simulink model "String3_Diode"  (R2023b)
settings: Solver=VariableStepAuto  StartTime=0.0  StopTime=1  FixedStep=Ts_Power  MinStep=0.0025  RelTol=1e-4
PreLoadFcn:
  | Ts_Power=5e-4;
  | Slope_Vdc=1;
InitFcn:
  | Ts_Power=50e-6;
  | Tc=1e-5;%break algebraic loop time constant
StopFcn:
  | if exist('I','var') && exist('V','var')
  |    figure(1)
  |    clf
  |    n=find(I>=0);
  |    n=n(end);
  |    Vglobal=V(1:n);
  |    Iglobal=I(1:n);
  | 
  | 
  |    Pglobal=Vglobal.*Iglobal;
  |    n=find(Pglobal==max(Pglobal));
  |    Pmax=Pglobal(n);
  |    Vmp=Vglobal(n);
  |    Imp=Iglobal(n);
  | 
  | 
  |    subplot(211)
  |    plot(Vglobal, Iglobal,Vmp,Imp,'or')
  |    ylabel('Current (A)')
  |    title(sprintf('Global I-V & P-V characteristics\n %s' ,ModuleName))
  | 
  | 
  |    subplot(212)
  |    plot(Vglobal, Pglobal,Vmp,Pmax,'or')
  |    ylabel('Power (W)')
  |    xlabel('Voltage (V)')
  | end
model workspace (MAT data in the model file):
  slope_Vdc = 3.0848387096
values from neighbouring files (symbols this model uses):
  Slope_Vdc_string3 = 90 * 0.77    (= 69.3)    [totPower.m]
libraries: spsPVArrayLib x90, spsVariableResistorLib x90, spsDiodeLib x20, spsCurrentMeasurementLib x1, spsVoltageMeasurementLib x1, spsControlledVoltageSourceLib x1, simulink x1, spspowerguiLib x1
(part 4 of 5)

== system String3_Diode/Subsystem17/PV10 ==
  Irr : Inport
  1PΩ : Constant  Value=1e15
  PV1 : spsPVArrayLib/PV Array  Npar=1  Nser=1  PlotType=array @ 25 deg.C & specified irradiances  S_vec="[ 1000  500  100 ]"  Temp_C_vec="[ 45 25  ]"  ModuleName=User-defined  PlotWhenSelected=off  Pm=3.8061  Ncell=1  Voc=0.7315  Isc=6.41  Vm=0.626  Im=6.08  beta_Voc_pc=-0.2256195755  alpha_Isc_pc=0.04692556634  beta_Voc=-0.0016504  alpha_Isc=0.0030079  IL=6.4137  I0=6.5578e-13  nI=0.95237  Rsh=7.312  Rs=0.0042689  RobustModel=on  RobustCellTemperature=25  BAL=on  Tc=1e-5  Tfilter=5e-5
  Terminator1 : Terminator
  Variable Resistor2 : spsVariableResistorLib/Variable Resistor  Rabsmin=1e-3
      settings: LibrarySourceBlock=sps_lib/Passives/Variable Resistor
  + : PMIOPort  Side=Left
  - : PMIOPort  Port=2  Side=Right
  wires:
  Irr/1 -> PV1/1
  1PΩ/1 -> Variable Resistor2/1
  PV1/1 -> Terminator1/1
  connections:
  PV1/RConn2 -- -/RConn1 -- Variable Resistor2/RConn1
  +/RConn1 -- Variable Resistor2/LConn1 -- PV1/RConn1

== system String3_Diode/Subsystem17/PV11 ==
  Irr : Inport
  1PΩ : Constant  Value=1e15
  PV2 : spsPVArrayLib/PV Array  Npar=1  Nser=1  PlotType=array @ 25 deg.C & specified irradiances  S_vec="[ 1000  500  100 ]"  Temp_C_vec="[ 45 25  ]"  ModuleName=User-defined  PlotWhenSelected=off  Pm=3.8061  Ncell=1  Voc=0.7315  Isc=6.41  Vm=0.626  Im=6.08  beta_Voc_pc=-0.2256195755  alpha_Isc_pc=0.04692556634  beta_Voc=-0.0016504  alpha_Isc=0.0030079  IL=6.4137  I0=6.5578e-13  nI=0.95237  Rsh=7.312  Rs=0.0042689  RobustModel=on  RobustCellTemperature=25  BAL=on  Tc=1e-5  Tfilter=5e-5
  Terminator1 : Terminator
  Variable Resistor2 : spsVariableResistorLib/Variable Resistor  Rabsmin=1e-3
      settings: LibrarySourceBlock=sps_lib/Passives/Variable Resistor
  + : PMIOPort  Side=Left
  - : PMIOPort  Port=2  Side=Right
  wires:
  Irr/1 -> PV2/1
  1PΩ/1 -> Variable Resistor2/1
  PV2/1 -> Terminator1/1
  connections:
  -/RConn1 -- Variable Resistor2/RConn1 -- PV2/RConn2
  +/RConn1 -- Variable Resistor2/LConn1 -- PV2/RConn1

== system String3_Diode/Subsystem17/PV2 ==
  Irr : Inport
  1PΩ : Constant  Value=1e15
  PV1 : spsPVArrayLib/PV Array  Npar=1  Nser=1  PlotType=array @ 25 deg.C & specified irradiances  S_vec="[ 1000  500  100 ]"  Temp_C_vec="[ 45 25  ]"  ModuleName=User-defined  PlotWhenSelected=off  Pm=3.8061  Ncell=1  Voc=0.7315  Isc=6.41  Vm=0.626  Im=6.08  beta_Voc_pc=-0.2256195755  alpha_Isc_pc=0.04692556634  beta_Voc=-0.0016504  alpha_Isc=0.0030079  IL=6.4137  I0=6.5578e-13  nI=0.95237  Rsh=7.312  Rs=0.0042689  RobustModel=on  RobustCellTemperature=25  BAL=on  Tc=1e-5  Tfilter=5e-5
  Terminator1 : Terminator
  Variable Resistor2 : spsVariableResistorLib/Variable Resistor  Rabsmin=1e-3
      settings: LibrarySourceBlock=sps_lib/Passives/Variable Resistor
  + : PMIOPort  Side=Left
  - : PMIOPort  Port=2  Side=Right
  wires:
  Irr/1 -> PV1/1
  1PΩ/1 -> Variable Resistor2/1
  PV1/1 -> Terminator1/1
  connections:
  PV1/RConn2 -- -/RConn1 -- Variable Resistor2/RConn1
  +/RConn1 -- Variable Resistor2/LConn1 -- PV1/RConn1

== system String3_Diode/Subsystem17/PV3 ==
  Irr : Inport
  1PΩ : Constant  Value=1e15
  PV1 : spsPVArrayLib/PV Array  Npar=1  Nser=1  PlotType=array @ 25 deg.C & specified irradiances  S_vec="[ 1000  500  100 ]"  Temp_C_vec="[ 45 25  ]"  ModuleName=User-defined  PlotWhenSelected=off  Pm=3.8061  Ncell=1  Voc=0.7315  Isc=6.41  Vm=0.626  Im=6.08  beta_Voc_pc=-0.2256195755  alpha_Isc_pc=0.04692556634  beta_Voc=-0.0016504  alpha_Isc=0.0030079  IL=6.4137  I0=6.5578e-13  nI=0.95237  Rsh=7.312  Rs=0.0042689  RobustModel=on  RobustCellTemperature=25  BAL=on  Tc=1e-5  Tfilter=5e-5
  Terminator1 : Terminator
  Variable Resistor2 : spsVariableResistorLib/Variable Resistor  Rabsmin=1e-3
      settings: LibrarySourceBlock=sps_lib/Passives/Variable Resistor
  + : PMIOPort  Side=Left
  - : PMIOPort  Port=2  Side=Right
  wires:
  Irr/1 -> PV1/1
  1PΩ/1 -> Variable Resistor2/1
  PV1/1 -> Terminator1/1
  connections:
  PV1/RConn2 -- -/RConn1 -- Variable Resistor2/RConn1
  +/RConn1 -- Variable Resistor2/LConn1 -- PV1/RConn1

== system String3_Diode/Subsystem18/PV1 ==
  Irr : Inport
  1PΩ : Constant  Value=1e15
  PV2 : spsPVArrayLib/PV Array  Npar=1  Nser=1  PlotType=array @ 25 deg.C & specified irradiances  S_vec="[ 1000  500  100 ]"  Temp_C_vec="[ 45 25  ]"  ModuleName=User-defined  PlotWhenSelected=off  Pm=3.8061  Ncell=1  Voc=0.7315  Isc=6.41  Vm=0.626  Im=6.08  beta_Voc_pc=-0.2256195755  alpha_Isc_pc=0.04692556634  beta_Voc=-0.0016504  alpha_Isc=0.0030079  IL=6.4137  I0=6.5578e-13  nI=0.95237  Rsh=7.312  Rs=0.0042689  RobustModel=on  RobustCellTemperature=25  BAL=on  Tc=1e-5  Tfilter=5e-5
  Terminator1 : Terminator
  Variable Resistor2 : spsVariableResistorLib/Variable Resistor  Rabsmin=1e-3
      settings: LibrarySourceBlock=sps_lib/Passives/Variable Resistor
  + : PMIOPort  Side=Left
  - : PMIOPort  Port=2  Side=Right
  wires:
  Irr/1 -> PV2/1
  1PΩ/1 -> Variable Resistor2/1
  PV2/1 -> Terminator1/1
  connections:
  -/RConn1 -- Variable Resistor2/RConn1 -- PV2/RConn2
  +/RConn1 -- Variable Resistor2/LConn1 -- PV2/RConn1

== system String3_Diode/Subsystem18/PV2 ==
  Irr : Inport
  1PΩ : Constant  Value=1e15
  PV2 : spsPVArrayLib/PV Array  Npar=1  Nser=1  PlotType=array @ 25 deg.C & specified irradiances  S_vec="[ 1000  500  100 ]"  Temp_C_vec="[ 45 25  ]"  ModuleName=User-defined  PlotWhenSelected=off  Pm=3.8061  Ncell=1  Voc=0.7315  Isc=6.41  Vm=0.626  Im=6.08  beta_Voc_pc=-0.2256195755  alpha_Isc_pc=0.04692556634  beta_Voc=-0.0016504  alpha_Isc=0.0030079  IL=6.4137  I0=6.5578e-13  nI=0.95237  Rsh=7.312  Rs=0.0042689  RobustModel=on  RobustCellTemperature=25  BAL=on  Tc=1e-5  Tfilter=5e-5
  Terminator1 : Terminator
  Variable Resistor2 : spsVariableResistorLib/Variable Resistor  Rabsmin=1e-3
      settings: LibrarySourceBlock=sps_lib/Passives/Variable Resistor
  + : PMIOPort  Side=Left
  - : PMIOPort  Port=2  Side=Right
  wires:
  Irr/1 -> PV2/1
  1PΩ/1 -> Variable Resistor2/1
  PV2/1 -> Terminator1/1
  connections:
  -/RConn1 -- Variable Resistor2/RConn1 -- PV2/RConn2
  +/RConn1 -- Variable Resistor2/LConn1 -- PV2/RConn1

== system String3_Diode/Subsystem18/PV3 ==
  Irr : Inport
  1PΩ : Constant  Value=1e15
  PV2 : spsPVArrayLib/PV Array  Npar=1  Nser=1  PlotType=array @ 25 deg.C & specified irradiances  S_vec="[ 1000  500  100 ]"  Temp_C_vec="[ 45 25  ]"  ModuleName=User-defined  PlotWhenSelected=off  Pm=3.8061  Ncell=1  Voc=0.7315  Isc=6.41  Vm=0.626  Im=6.08  beta_Voc_pc=-0.2256195755  alpha_Isc_pc=0.04692556634  beta_Voc=-0.0016504  alpha_Isc=0.0030079  IL=6.4137  I0=6.5578e-13  nI=0.95237  Rsh=7.312  Rs=0.0042689  RobustModel=on  RobustCellTemperature=25  BAL=on  Tc=1e-5  Tfilter=5e-5
  Terminator1 : Terminator
  Variable Resistor2 : spsVariableResistorLib/Variable Resistor  Rabsmin=1e-3
      settings: LibrarySourceBlock=sps_lib/Passives/Variable Resistor
  + : PMIOPort  Side=Left
  - : PMIOPort  Port=2  Side=Right
  wires:
  Irr/1 -> PV2/1
  1PΩ/1 -> Variable Resistor2/1
  PV2/1 -> Terminator1/1
  connections:
  -/RConn1 -- PV2/RConn2 -- Variable Resistor2/RConn1
  +/RConn1 -- PV2/RConn1 -- Variable Resistor2/LConn1

== system String3_Diode/Subsystem18/PV4 ==
  Irr : Inport
  1PΩ : Constant  Value=1e15
  PV2 : spsPVArrayLib/PV Array  Npar=1  Nser=1  PlotType=array @ 25 deg.C & specified irradiances  S_vec="[ 1000  500  100 ]"  Temp_C_vec="[ 45 25  ]"  ModuleName=User-defined  PlotWhenSelected=off  Pm=3.8061  Ncell=1  Voc=0.7315  Isc=6.41  Vm=0.626  Im=6.08  beta_Voc_pc=-0.2256195755  alpha_Isc_pc=0.04692556634  beta_Voc=-0.0016504  alpha_Isc=0.0030079  IL=6.4137  I0=6.5578e-13  nI=0.95237  Rsh=7.312  Rs=0.0042689  RobustModel=on  RobustCellTemperature=25  BAL=on  Tc=1e-5  Tfilter=5e-5
  Terminator1 : Terminator
  Variable Resistor2 : spsVariableResistorLib/Variable Resistor  Rabsmin=1e-3
      settings: LibrarySourceBlock=sps_lib/Passives/Variable Resistor
  + : PMIOPort  Side=Left
  - : PMIOPort  Port=2  Side=Right
  wires:
  Irr/1 -> PV2/1
  1PΩ/1 -> Variable Resistor2/1
  PV2/1 -> Terminator1/1
  connections:
  -/RConn1 -- Variable Resistor2/RConn1 -- PV2/RConn2
  +/RConn1 -- Variable Resistor2/LConn1 -- PV2/RConn1

== system String3_Diode/Subsystem19/PV1 ==
  Irr : Inport
  1PΩ : Constant  Value=1e15
  PV2 : spsPVArrayLib/PV Array  Npar=1  Nser=1  PlotType=array @ 25 deg.C & specified irradiances  S_vec="[ 1000  500  100 ]"  Temp_C_vec="[ 45 25  ]"  ModuleName=User-defined  PlotWhenSelected=off  Pm=3.8061  Ncell=1  Voc=0.7315  Isc=6.41  Vm=0.626  Im=6.08  beta_Voc_pc=-0.2256195755  alpha_Isc_pc=0.04692556634  beta_Voc=-0.0016504  alpha_Isc=0.0030079  IL=6.4137  I0=6.5578e-13  nI=0.95237  Rsh=7.312  Rs=0.0042689  RobustModel=on  RobustCellTemperature=25  BAL=on  Tc=1e-5  Tfilter=5e-5
  Terminator1 : Terminator
  Variable Resistor2 : spsVariableResistorLib/Variable Resistor  Rabsmin=1e-3
      settings: LibrarySourceBlock=sps_lib/Passives/Variable Resistor
  + : PMIOPort  Side=Left
  - : PMIOPort  Port=2  Side=Right
  wires:
  Irr/1 -> PV2/1
  1PΩ/1 -> Variable Resistor2/1
  PV2/1 -> Terminator1/1
  connections:
  -/RConn1 -- Variable Resistor2/RConn1 -- PV2/RConn2
  +/RConn1 -- Variable Resistor2/LConn1 -- PV2/RConn1

== system String3_Diode/Subsystem19/PV2 ==
  Irr : Inport
  1PΩ : Constant  Value=1e15
  PV2 : spsPVArrayLib/PV Array  Npar=1  Nser=1  PlotType=array @ 25 deg.C & specified irradiances  S_vec="[ 1000  500  100 ]"  Temp_C_vec="[ 45 25  ]"  ModuleName=User-defined  PlotWhenSelected=off  Pm=3.8061  Ncell=1  Voc=0.7315  Isc=6.41  Vm=0.626  Im=6.08  beta_Voc_pc=-0.2256195755  alpha_Isc_pc=0.04692556634  beta_Voc=-0.0016504  alpha_Isc=0.0030079  IL=6.4137  I0=6.5578e-13  nI=0.95237  Rsh=7.312  Rs=0.0042689  RobustModel=on  RobustCellTemperature=25  BAL=on  Tc=1e-5  Tfilter=5e-5
  Terminator1 : Terminator
  Variable Resistor2 : spsVariableResistorLib/Variable Resistor  Rabsmin=1e-3
      settings: LibrarySourceBlock=sps_lib/Passives/Variable Resistor
  + : PMIOPort  Side=Left
  - : PMIOPort  Port=2  Side=Right
  wires:
  Irr/1 -> PV2/1
  1PΩ/1 -> Variable Resistor2/1
  PV2/1 -> Terminator1/1
  connections:
  -/RConn1 -- Variable Resistor2/RConn1 -- PV2/RConn2
  +/RConn1 -- Variable Resistor2/LConn1 -- PV2/RConn1

== system String3_Diode/Subsystem19/PV3 ==
  Irr : Inport
  1PΩ : Constant  Value=1e15
  PV2 : spsPVArrayLib/PV Array  Npar=1  Nser=1  PlotType=array @ 25 deg.C & specified irradiances  S_vec="[ 1000  500  100 ]"  Temp_C_vec="[ 45 25  ]"  ModuleName=User-defined  PlotWhenSelected=off  Pm=3.8061  Ncell=1  Voc=0.7315  Isc=6.41  Vm=0.626  Im=6.08  beta_Voc_pc=-0.2256195755  alpha_Isc_pc=0.04692556634  beta_Voc=-0.0016504  alpha_Isc=0.0030079  IL=6.4137  I0=6.5578e-13  nI=0.95237  Rsh=7.312  Rs=0.0042689  RobustModel=on  RobustCellTemperature=25  BAL=on  Tc=1e-5  Tfilter=5e-5
  Terminator1 : Terminator
  Variable Resistor2 : spsVariableResistorLib/Variable Resistor  Rabsmin=1e-3
      settings: LibrarySourceBlock=sps_lib/Passives/Variable Resistor
  + : PMIOPort  Side=Left
  - : PMIOPort  Port=2  Side=Right
  wires:
  Irr/1 -> PV2/1
  1PΩ/1 -> Variable Resistor2/1
  PV2/1 -> Terminator1/1
  connections:
  -/RConn1 -- PV2/RConn2 -- Variable Resistor2/RConn1
  +/RConn1 -- PV2/RConn1 -- Variable Resistor2/LConn1

== system String3_Diode/Subsystem19/PV4 ==
  Irr : Inport
  1PΩ : Constant  Value=1e15
  PV2 : spsPVArrayLib/PV Array  Npar=1  Nser=1  PlotType=array @ 25 deg.C & specified irradiances  S_vec="[ 1000  500  100 ]"  Temp_C_vec="[ 45 25  ]"  ModuleName=User-defined  PlotWhenSelected=off  Pm=3.8061  Ncell=1  Voc=0.7315  Isc=6.41  Vm=0.626  Im=6.08  beta_Voc_pc=-0.2256195755  alpha_Isc_pc=0.04692556634  beta_Voc=-0.0016504  alpha_Isc=0.0030079  IL=6.4137  I0=6.5578e-13  nI=0.95237  Rsh=7.312  Rs=0.0042689  RobustModel=on  RobustCellTemperature=25  BAL=on  Tc=1e-5  Tfilter=5e-5
  Terminator1 : Terminator
  Variable Resistor2 : spsVariableResistorLib/Variable Resistor  Rabsmin=1e-3
      settings: LibrarySourceBlock=sps_lib/Passives/Variable Resistor
  + : PMIOPort  Side=Left
  - : PMIOPort  Port=2  Side=Right
  wires:
  Irr/1 -> PV2/1
  1PΩ/1 -> Variable Resistor2/1
  PV2/1 -> Terminator1/1
  connections:
  -/RConn1 -- Variable Resistor2/RConn1 -- PV2/RConn2
  +/RConn1 -- Variable Resistor2/LConn1 -- PV2/RConn1

== system String3_Diode/Subsystem20/PV1 ==
  Irr : Inport
  1PΩ : Constant  Value=1e15
  PV2 : spsPVArrayLib/PV Array  Npar=1  Nser=1  PlotType=array @ 25 deg.C & specified irradiances  S_vec="[ 1000  500  100 ]"  Temp_C_vec="[ 45 25  ]"  ModuleName=User-defined  PlotWhenSelected=off  Pm=3.8061  Ncell=1  Voc=0.7315  Isc=6.41  Vm=0.626  Im=6.08  beta_Voc_pc=-0.2256195755  alpha_Isc_pc=0.04692556634  beta_Voc=-0.0016504  alpha_Isc=0.0030079  IL=6.4137  I0=6.5578e-13  nI=0.95237  Rsh=7.312  Rs=0.0042689  RobustModel=on  RobustCellTemperature=25  BAL=on  Tc=1e-5  Tfilter=5e-5
  Terminator1 : Terminator
  Variable Resistor2 : spsVariableResistorLib/Variable Resistor  Rabsmin=1e-3
      settings: LibrarySourceBlock=sps_lib/Passives/Variable Resistor
  + : PMIOPort  Side=Left
  - : PMIOPort  Port=2  Side=Right
  wires:
  Irr/1 -> PV2/1
  1PΩ/1 -> Variable Resistor2/1
  PV2/1 -> Terminator1/1
  connections:
  -/RConn1 -- Variable Resistor2/RConn1 -- PV2/RConn2
  +/RConn1 -- Variable Resistor2/LConn1 -- PV2/RConn1

== system String3_Diode/Subsystem20/PV2 ==
  Irr : Inport
  1PΩ : Constant  Value=1e15
  PV2 : spsPVArrayLib/PV Array  Npar=1  Nser=1  PlotType=array @ 25 deg.C & specified irradiances  S_vec="[ 1000  500  100 ]"  Temp_C_vec="[ 45 25  ]"  ModuleName=User-defined  PlotWhenSelected=off  Pm=3.8061  Ncell=1  Voc=0.7315  Isc=6.41  Vm=0.626  Im=6.08  beta_Voc_pc=-0.2256195755  alpha_Isc_pc=0.04692556634  beta_Voc=-0.0016504  alpha_Isc=0.0030079  IL=6.4137  I0=6.5578e-13  nI=0.95237  Rsh=7.312  Rs=0.0042689  RobustModel=on  RobustCellTemperature=25  BAL=on  Tc=1e-5  Tfilter=5e-5
  Terminator1 : Terminator
  Variable Resistor2 : spsVariableResistorLib/Variable Resistor  Rabsmin=1e-3
      settings: LibrarySourceBlock=sps_lib/Passives/Variable Resistor
  + : PMIOPort  Side=Left
  - : PMIOPort  Port=2  Side=Right
  wires:
  Irr/1 -> PV2/1
  1PΩ/1 -> Variable Resistor2/1
  PV2/1 -> Terminator1/1
  connections:
  -/RConn1 -- Variable Resistor2/RConn1 -- PV2/RConn2
  +/RConn1 -- Variable Resistor2/LConn1 -- PV2/RConn1

== system String3_Diode/Subsystem20/PV3 ==
  Irr : Inport
  1PΩ : Constant  Value=1e15
  PV2 : spsPVArrayLib/PV Array  Npar=1  Nser=1  PlotType=array @ 25 deg.C & specified irradiances  S_vec="[ 1000  500  100 ]"  Temp_C_vec="[ 45 25  ]"  ModuleName=User-defined  PlotWhenSelected=off  Pm=3.8061  Ncell=1  Voc=0.7315  Isc=6.41  Vm=0.626  Im=6.08  beta_Voc_pc=-0.2256195755  alpha_Isc_pc=0.04692556634  beta_Voc=-0.0016504  alpha_Isc=0.0030079  IL=6.4137  I0=6.5578e-13  nI=0.95237  Rsh=7.312  Rs=0.0042689  RobustModel=on  RobustCellTemperature=25  BAL=on  Tc=1e-5  Tfilter=5e-5
  Terminator1 : Terminator
  Variable Resistor2 : spsVariableResistorLib/Variable Resistor  Rabsmin=1e-3
      settings: LibrarySourceBlock=sps_lib/Passives/Variable Resistor
  + : PMIOPort  Side=Left
  - : PMIOPort  Port=2  Side=Right
  wires:
  Irr/1 -> PV2/1
  1PΩ/1 -> Variable Resistor2/1
  PV2/1 -> Terminator1/1
  connections:
  -/RConn1 -- PV2/RConn2 -- Variable Resistor2/RConn1
  +/RConn1 -- PV2/RConn1 -- Variable Resistor2/LConn1

== system String3_Diode/Subsystem20/PV4 ==
  Irr : Inport
  1PΩ : Constant  Value=1e15
  PV2 : spsPVArrayLib/PV Array  Npar=1  Nser=1  PlotType=array @ 25 deg.C & specified irradiances  S_vec="[ 1000  500  100 ]"  Temp_C_vec="[ 45 25  ]"  ModuleName=User-defined  PlotWhenSelected=off  Pm=3.8061  Ncell=1  Voc=0.7315  Isc=6.41  Vm=0.626  Im=6.08  beta_Voc_pc=-0.2256195755  alpha_Isc_pc=0.04692556634  beta_Voc=-0.0016504  alpha_Isc=0.0030079  IL=6.4137  I0=6.5578e-13  nI=0.95237  Rsh=7.312  Rs=0.0042689  RobustModel=on  RobustCellTemperature=25  BAL=on  Tc=1e-5  Tfilter=5e-5
  Terminator1 : Terminator
  Variable Resistor2 : spsVariableResistorLib/Variable Resistor  Rabsmin=1e-3
      settings: LibrarySourceBlock=sps_lib/Passives/Variable Resistor
  + : PMIOPort  Side=Left
  - : PMIOPort  Port=2  Side=Right
  wires:
  Irr/1 -> PV2/1
  1PΩ/1 -> Variable Resistor2/1
  PV2/1 -> Terminator1/1
  connections:
  -/RConn1 -- Variable Resistor2/RConn1 -- PV2/RConn2
  +/RConn1 -- Variable Resistor2/LConn1 -- PV2/RConn1

== system String3_Diode/Subsystem25/PV1 ==
  Irr : Inport
  1PΩ : Constant  Value=1e15
  PV2 : spsPVArrayLib/PV Array  Npar=1  Nser=1  PlotType=array @ 25 deg.C & specified irradiances  S_vec="[ 1000  500  100 ]"  Temp_C_vec="[ 45 25  ]"  ModuleName=User-defined  PlotWhenSelected=off  Pm=3.8061  Ncell=1  Voc=0.7315  Isc=6.41  Vm=0.626  Im=6.08  beta_Voc_pc=-0.2256195755  alpha_Isc_pc=0.04692556634  beta_Voc=-0.0016504  alpha_Isc=0.0030079  IL=6.4137  I0=6.5578e-13  nI=0.95237  Rsh=7.312  Rs=0.0042689  RobustModel=on  RobustCellTemperature=25  BAL=on  Tc=1e-5  Tfilter=5e-5
  Terminator1 : Terminator
  Variable Resistor2 : spsVariableResistorLib/Variable Resistor  Rabsmin=1e-3
      settings: LibrarySourceBlock=sps_lib/Passives/Variable Resistor
  + : PMIOPort  Side=Left
  - : PMIOPort  Port=2  Side=Right
  wires:
  Irr/1 -> PV2/1
  1PΩ/1 -> Variable Resistor2/1
  PV2/1 -> Terminator1/1
  connections:
  -/RConn1 -- Variable Resistor2/RConn1 -- PV2/RConn2
  +/RConn1 -- Variable Resistor2/LConn1 -- PV2/RConn1

== system String3_Diode/Subsystem25/PV2 ==
  Irr : Inport
  1PΩ : Constant  Value=1e15
  PV2 : spsPVArrayLib/PV Array  Npar=1  Nser=1  PlotType=array @ 25 deg.C & specified irradiances  S_vec="[ 1000  500  100 ]"  Temp_C_vec="[ 45 25  ]"  ModuleName=User-defined  PlotWhenSelected=off  Pm=3.8061  Ncell=1  Voc=0.7315  Isc=6.41  Vm=0.626  Im=6.08  beta_Voc_pc=-0.2256195755  alpha_Isc_pc=0.04692556634  beta_Voc=-0.0016504  alpha_Isc=0.0030079  IL=6.4137  I0=6.5578e-13  nI=0.95237  Rsh=7.312  Rs=0.0042689  RobustModel=on  RobustCellTemperature=25  BAL=on  Tc=1e-5  Tfilter=5e-5
  Terminator1 : Terminator
  Variable Resistor2 : spsVariableResistorLib/Variable Resistor  Rabsmin=1e-3
      settings: LibrarySourceBlock=sps_lib/Passives/Variable Resistor
  + : PMIOPort  Side=Left
  - : PMIOPort  Port=2  Side=Right
  wires:
  Irr/1 -> PV2/1
  1PΩ/1 -> Variable Resistor2/1
  PV2/1 -> Terminator1/1
  connections:
  -/RConn1 -- Variable Resistor2/RConn1 -- PV2/RConn2
  +/RConn1 -- Variable Resistor2/LConn1 -- PV2/RConn1

== system String3_Diode/Subsystem25/PV3 ==
  Irr : Inport
  1PΩ : Constant  Value=1e15
  PV2 : spsPVArrayLib/PV Array  Npar=1  Nser=1  PlotType=array @ 25 deg.C & specified irradiances  S_vec="[ 1000  500  100 ]"  Temp_C_vec="[ 45 25  ]"  ModuleName=User-defined  PlotWhenSelected=off  Pm=3.8061  Ncell=1  Voc=0.7315  Isc=6.41  Vm=0.626  Im=6.08  beta_Voc_pc=-0.2256195755  alpha_Isc_pc=0.04692556634  beta_Voc=-0.0016504  alpha_Isc=0.0030079  IL=6.4137  I0=6.5578e-13  nI=0.95237  Rsh=7.312  Rs=0.0042689  RobustModel=on  RobustCellTemperature=25  BAL=on  Tc=1e-5  Tfilter=5e-5
  Terminator1 : Terminator
  Variable Resistor2 : spsVariableResistorLib/Variable Resistor  Rabsmin=1e-3
      settings: LibrarySourceBlock=sps_lib/Passives/Variable Resistor
  + : PMIOPort  Side=Left
  - : PMIOPort  Port=2  Side=Right
  wires:
  Irr/1 -> PV2/1
  1PΩ/1 -> Variable Resistor2/1
  PV2/1 -> Terminator1/1
  connections:
  -/RConn1 -- PV2/RConn2 -- Variable Resistor2/RConn1
  +/RConn1 -- PV2/RConn1 -- Variable Resistor2/LConn1

== system String3_Diode/Subsystem25/PV4 ==
  Irr : Inport
  1PΩ : Constant  Value=1e15
  PV2 : spsPVArrayLib/PV Array  Npar=1  Nser=1  PlotType=array @ 25 deg.C & specified irradiances  S_vec="[ 1000  500  100 ]"  Temp_C_vec="[ 45 25  ]"  ModuleName=User-defined  PlotWhenSelected=off  Pm=3.8061  Ncell=1  Voc=0.7315  Isc=6.41  Vm=0.626  Im=6.08  beta_Voc_pc=-0.2256195755  alpha_Isc_pc=0.04692556634  beta_Voc=-0.0016504  alpha_Isc=0.0030079  IL=6.4137  I0=6.5578e-13  nI=0.95237  Rsh=7.312  Rs=0.0042689  RobustModel=on  RobustCellTemperature=25  BAL=on  Tc=1e-5  Tfilter=5e-5
  Terminator1 : Terminator
  Variable Resistor2 : spsVariableResistorLib/Variable Resistor  Rabsmin=1e-3
      settings: LibrarySourceBlock=sps_lib/Passives/Variable Resistor
  + : PMIOPort  Side=Left
  - : PMIOPort  Port=2  Side=Right
  wires:
  Irr/1 -> PV2/1
  1PΩ/1 -> Variable Resistor2/1
  PV2/1 -> Terminator1/1
  connections:
  -/RConn1 -- Variable Resistor2/RConn1 -- PV2/RConn2
  +/RConn1 -- Variable Resistor2/LConn1 -- PV2/RConn1

== system String3_Diode/Subsystem3/PV1 ==
  Irr : Inport
  1PΩ : Constant  Value=1e15
  PV2 : spsPVArrayLib/PV Array  Npar=1  Nser=1  PlotType=array @ 25 deg.C & specified irradiances  S_vec="[ 1000  500  100 ]"  Temp_C_vec="[ 45 25  ]"  ModuleName=User-defined  PlotWhenSelected=off  Pm=3.8061  Ncell=1  Voc=0.7315  Isc=6.41  Vm=0.626  Im=6.08  beta_Voc_pc=-0.2256195755  alpha_Isc_pc=0.04692556634  beta_Voc=-0.0016504  alpha_Isc=0.0030079  IL=6.4137  I0=6.5578e-13  nI=0.95237  Rsh=7.312  Rs=0.0042689  RobustModel=on  RobustCellTemperature=25  BAL=on  Tc=1e-5  Tfilter=5e-5
  Terminator1 : Terminator
  Variable Resistor2 : spsVariableResistorLib/Variable Resistor  Rabsmin=1e-3
      settings: LibrarySourceBlock=sps_lib/Passives/Variable Resistor
  + : PMIOPort  Side=Left
  - : PMIOPort  Port=2  Side=Right
  wires:
  Irr/1 -> PV2/1
  1PΩ/1 -> Variable Resistor2/1
  PV2/1 -> Terminator1/1
  connections:
  -/RConn1 -- Variable Resistor2/RConn1 -- PV2/RConn2
  +/RConn1 -- Variable Resistor2/LConn1 -- PV2/RConn1

== system String3_Diode/Subsystem3/PV2 ==
  Irr : Inport
  1PΩ : Constant  Value=1e15
  PV2 : spsPVArrayLib/PV Array  Npar=1  Nser=1  PlotType=array @ 25 deg.C & specified irradiances  S_vec="[ 1000  500  100 ]"  Temp_C_vec="[ 45 25  ]"  ModuleName=User-defined  PlotWhenSelected=off  Pm=3.8061  Ncell=1  Voc=0.7315  Isc=6.41  Vm=0.626  Im=6.08  beta_Voc_pc=-0.2256195755  alpha_Isc_pc=0.04692556634  beta_Voc=-0.0016504  alpha_Isc=0.0030079  IL=6.4137  I0=6.5578e-13  nI=0.95237  Rsh=7.312  Rs=0.0042689  RobustModel=on  RobustCellTemperature=25  BAL=on  Tc=1e-5  Tfilter=5e-5
  Terminator1 : Terminator
  Variable Resistor2 : spsVariableResistorLib/Variable Resistor  Rabsmin=1e-3
      settings: LibrarySourceBlock=sps_lib/Passives/Variable Resistor
  + : PMIOPort  Side=Left
  - : PMIOPort  Port=2  Side=Right
  wires:
  Irr/1 -> PV2/1
  1PΩ/1 -> Variable Resistor2/1
  PV2/1 -> Terminator1/1
  connections:
  -/RConn1 -- Variable Resistor2/RConn1 -- PV2/RConn2
  +/RConn1 -- Variable Resistor2/LConn1 -- PV2/RConn1

== system String3_Diode/Subsystem3/PV3 ==
  Irr : Inport
  1PΩ : Constant  Value=1e15
  PV2 : spsPVArrayLib/PV Array  Npar=1  Nser=1  PlotType=array @ 25 deg.C & specified irradiances  S_vec="[ 1000  500  100 ]"  Temp_C_vec="[ 45 25  ]"  ModuleName=User-defined  PlotWhenSelected=off  Pm=3.8061  Ncell=1  Voc=0.7315  Isc=6.41  Vm=0.626  Im=6.08  beta_Voc_pc=-0.2256195755  alpha_Isc_pc=0.04692556634  beta_Voc=-0.0016504  alpha_Isc=0.0030079  IL=6.4137  I0=6.5578e-13  nI=0.95237  Rsh=7.312  Rs=0.0042689  RobustModel=on  RobustCellTemperature=25  BAL=on  Tc=1e-5  Tfilter=5e-5
  Terminator1 : Terminator
  Variable Resistor2 : spsVariableResistorLib/Variable Resistor  Rabsmin=1e-3
      settings: LibrarySourceBlock=sps_lib/Passives/Variable Resistor
  + : PMIOPort  Side=Left
  - : PMIOPort  Port=2  Side=Right
  wires:
  Irr/1 -> PV2/1
  1PΩ/1 -> Variable Resistor2/1
  PV2/1 -> Terminator1/1
  connections:
  -/RConn1 -- PV2/RConn2 -- Variable Resistor2/RConn1
  +/RConn1 -- PV2/RConn1 -- Variable Resistor2/LConn1

== system String3_Diode/Subsystem3/PV4 ==
  Irr : Inport
  1PΩ : Constant  Value=1e15
  PV2 : spsPVArrayLib/PV Array  Npar=1  Nser=1  PlotType=array @ 25 deg.C & specified irradiances  S_vec="[ 1000  500  100 ]"  Temp_C_vec="[ 45 25  ]"  ModuleName=User-defined  PlotWhenSelected=off  Pm=3.8061  Ncell=1  Voc=0.7315  Isc=6.41  Vm=0.626  Im=6.08  beta_Voc_pc=-0.2256195755  alpha_Isc_pc=0.04692556634  beta_Voc=-0.0016504  alpha_Isc=0.0030079  IL=6.4137  I0=6.5578e-13  nI=0.95237  Rsh=7.312  Rs=0.0042689  RobustModel=on  RobustCellTemperature=25  BAL=on  Tc=1e-5  Tfilter=5e-5
  Terminator1 : Terminator
  Variable Resistor2 : spsVariableResistorLib/Variable Resistor  Rabsmin=1e-3
      settings: LibrarySourceBlock=sps_lib/Passives/Variable Resistor
  + : PMIOPort  Side=Left
  - : PMIOPort  Port=2  Side=Right
  wires:
  Irr/1 -> PV2/1
  1PΩ/1 -> Variable Resistor2/1
  PV2/1 -> Terminator1/1
  connections:
  -/RConn1 -- Variable Resistor2/RConn1 -- PV2/RConn2
  +/RConn1 -- Variable Resistor2/LConn1 -- PV2/RConn1

== system String3_Diode/Subsystem35/PV1 ==
  Irr : Inport
  1PΩ : Constant  Value=1e15
  PV2 : spsPVArrayLib/PV Array  Npar=1  Nser=1  PlotType=array @ 25 deg.C & specified irradiances  S_vec="[ 1000  500  100 ]"  Temp_C_vec="[ 45 25  ]"  ModuleName=User-defined  PlotWhenSelected=off  Pm=3.8061  Ncell=1  Voc=0.7315  Isc=6.41  Vm=0.626  Im=6.08  beta_Voc_pc=-0.2256195755  alpha_Isc_pc=0.04692556634  beta_Voc=-0.0016504  alpha_Isc=0.0030079  IL=6.4137  I0=6.5578e-13  nI=0.95237  Rsh=7.312  Rs=0.0042689  RobustModel=on  RobustCellTemperature=25  BAL=on  Tc=1e-5  Tfilter=5e-5
  Terminator1 : Terminator
  Variable Resistor2 : spsVariableResistorLib/Variable Resistor  Rabsmin=1e-3
      settings: LibrarySourceBlock=sps_lib/Passives/Variable Resistor
  + : PMIOPort  Side=Left
  - : PMIOPort  Port=2  Side=Right
  wires:
  Irr/1 -> PV2/1
  1PΩ/1 -> Variable Resistor2/1
  PV2/1 -> Terminator1/1
  connections:
  -/RConn1 -- Variable Resistor2/RConn1 -- PV2/RConn2
  +/RConn1 -- Variable Resistor2/LConn1 -- PV2/RConn1

== system String3_Diode/Subsystem35/PV2 ==
  Irr : Inport
  1PΩ : Constant  Value=1e15
  PV2 : spsPVArrayLib/PV Array  Npar=1  Nser=1  PlotType=array @ 25 deg.C & specified irradiances  S_vec="[ 1000  500  100 ]"  Temp_C_vec="[ 45 25  ]"  ModuleName=User-defined  PlotWhenSelected=off  Pm=3.8061  Ncell=1  Voc=0.7315  Isc=6.41  Vm=0.626  Im=6.08  beta_Voc_pc=-0.2256195755  alpha_Isc_pc=0.04692556634  beta_Voc=-0.0016504  alpha_Isc=0.0030079  IL=6.4137  I0=6.5578e-13  nI=0.95237  Rsh=7.312  Rs=0.0042689  RobustModel=on  RobustCellTemperature=25  BAL=on  Tc=1e-5  Tfilter=5e-5
  Terminator1 : Terminator
  Variable Resistor2 : spsVariableResistorLib/Variable Resistor  Rabsmin=1e-3
      settings: LibrarySourceBlock=sps_lib/Passives/Variable Resistor
  + : PMIOPort  Side=Left
  - : PMIOPort  Port=2  Side=Right
  wires:
  Irr/1 -> PV2/1
  1PΩ/1 -> Variable Resistor2/1
  PV2/1 -> Terminator1/1
  connections:
  -/RConn1 -- Variable Resistor2/RConn1 -- PV2/RConn2
  +/RConn1 -- Variable Resistor2/LConn1 -- PV2/RConn1

== system String3_Diode/Subsystem35/PV3 ==
  Irr : Inport
  1PΩ : Constant  Value=1e15
  PV2 : spsPVArrayLib/PV Array  Npar=1  Nser=1  PlotType=array @ 25 deg.C & specified irradiances  S_vec="[ 1000  500  100 ]"  Temp_C_vec="[ 45 25  ]"  ModuleName=User-defined  PlotWhenSelected=off  Pm=3.8061  Ncell=1  Voc=0.7315  Isc=6.41  Vm=0.626  Im=6.08  beta_Voc_pc=-0.2256195755  alpha_Isc_pc=0.04692556634  beta_Voc=-0.0016504  alpha_Isc=0.0030079  IL=6.4137  I0=6.5578e-13  nI=0.95237  Rsh=7.312  Rs=0.0042689  RobustModel=on  RobustCellTemperature=25  BAL=on  Tc=1e-5  Tfilter=5e-5
  Terminator1 : Terminator
  Variable Resistor2 : spsVariableResistorLib/Variable Resistor  Rabsmin=1e-3
      settings: LibrarySourceBlock=sps_lib/Passives/Variable Resistor
  + : PMIOPort  Side=Left
  - : PMIOPort  Port=2  Side=Right
  wires:
  Irr/1 -> PV2/1
  1PΩ/1 -> Variable Resistor2/1
  PV2/1 -> Terminator1/1
  connections:
  -/RConn1 -- PV2/RConn2 -- Variable Resistor2/RConn1
  +/RConn1 -- PV2/RConn1 -- Variable Resistor2/LConn1

== system String3_Diode/Subsystem35/PV4 ==
  Irr : Inport
  1PΩ : Constant  Value=1e15
  PV2 : spsPVArrayLib/PV Array  Npar=1  Nser=1  PlotType=array @ 25 deg.C & specified irradiances  S_vec="[ 1000  500  100 ]"  Temp_C_vec="[ 45 25  ]"  ModuleName=User-defined  PlotWhenSelected=off  Pm=3.8061  Ncell=1  Voc=0.7315  Isc=6.41  Vm=0.626  Im=6.08  beta_Voc_pc=-0.2256195755  alpha_Isc_pc=0.04692556634  beta_Voc=-0.0016504  alpha_Isc=0.0030079  IL=6.4137  I0=6.5578e-13  nI=0.95237  Rsh=7.312  Rs=0.0042689  RobustModel=on  RobustCellTemperature=25  BAL=on  Tc=1e-5  Tfilter=5e-5
  Terminator1 : Terminator
  Variable Resistor2 : spsVariableResistorLib/Variable Resistor  Rabsmin=1e-3
      settings: LibrarySourceBlock=sps_lib/Passives/Variable Resistor
  + : PMIOPort  Side=Left
  - : PMIOPort  Port=2  Side=Right
  wires:
  Irr/1 -> PV2/1
  1PΩ/1 -> Variable Resistor2/1
  PV2/1 -> Terminator1/1
  connections:
  -/RConn1 -- Variable Resistor2/RConn1 -- PV2/RConn2
  +/RConn1 -- Variable Resistor2/LConn1 -- PV2/RConn1

== system String3_Diode/Subsystem36/PV1 ==
  Irr : Inport
  1PΩ : Constant  Value=1e15
  PV2 : spsPVArrayLib/PV Array  Npar=1  Nser=1  PlotType=array @ 25 deg.C & specified irradiances  S_vec="[ 1000  500  100 ]"  Temp_C_vec="[ 45 25  ]"  ModuleName=User-defined  PlotWhenSelected=off  Pm=3.8061  Ncell=1  Voc=0.7315  Isc=6.41  Vm=0.626  Im=6.08  beta_Voc_pc=-0.2256195755  alpha_Isc_pc=0.04692556634  beta_Voc=-0.0016504  alpha_Isc=0.0030079  IL=6.4137  I0=6.5578e-13  nI=0.95237  Rsh=7.312  Rs=0.0042689  RobustModel=on  RobustCellTemperature=25  BAL=on  Tc=1e-5  Tfilter=5e-5
  Terminator1 : Terminator
  Variable Resistor2 : spsVariableResistorLib/Variable Resistor  Rabsmin=1e-3
      settings: LibrarySourceBlock=sps_lib/Passives/Variable Resistor
  + : PMIOPort  Side=Left
  - : PMIOPort  Port=2  Side=Right
  wires:
  Irr/1 -> PV2/1
  1PΩ/1 -> Variable Resistor2/1
  PV2/1 -> Terminator1/1
  connections:
  -/RConn1 -- Variable Resistor2/RConn1 -- PV2/RConn2
  +/RConn1 -- Variable Resistor2/LConn1 -- PV2/RConn1

== system String3_Diode/Subsystem36/PV2 ==
  Irr : Inport
  1PΩ : Constant  Value=1e15
  PV2 : spsPVArrayLib/PV Array  Npar=1  Nser=1  PlotType=array @ 25 deg.C & specified irradiances  S_vec="[ 1000  500  100 ]"  Temp_C_vec="[ 45 25  ]"  ModuleName=User-defined  PlotWhenSelected=off  Pm=3.8061  Ncell=1  Voc=0.7315  Isc=6.41  Vm=0.626  Im=6.08  beta_Voc_pc=-0.2256195755  alpha_Isc_pc=0.04692556634  beta_Voc=-0.0016504  alpha_Isc=0.0030079  IL=6.4137  I0=6.5578e-13  nI=0.95237  Rsh=7.312  Rs=0.0042689  RobustModel=on  RobustCellTemperature=25  BAL=on  Tc=1e-5  Tfilter=5e-5
  Terminator1 : Terminator
  Variable Resistor2 : spsVariableResistorLib/Variable Resistor  Rabsmin=1e-3
      settings: LibrarySourceBlock=sps_lib/Passives/Variable Resistor
  + : PMIOPort  Side=Left
  - : PMIOPort  Port=2  Side=Right
  wires:
  Irr/1 -> PV2/1
  1PΩ/1 -> Variable Resistor2/1
  PV2/1 -> Terminator1/1
  connections:
  -/RConn1 -- Variable Resistor2/RConn1 -- PV2/RConn2
  +/RConn1 -- Variable Resistor2/LConn1 -- PV2/RConn1

== system String3_Diode/Subsystem36/PV3 ==
  Irr : Inport
  1PΩ : Constant  Value=1e15
  PV2 : spsPVArrayLib/PV Array  Npar=1  Nser=1  PlotType=array @ 25 deg.C & specified irradiances  S_vec="[ 1000  500  100 ]"  Temp_C_vec="[ 45 25  ]"  ModuleName=User-defined  PlotWhenSelected=off  Pm=3.8061  Ncell=1  Voc=0.7315  Isc=6.41  Vm=0.626  Im=6.08  beta_Voc_pc=-0.2256195755  alpha_Isc_pc=0.04692556634  beta_Voc=-0.0016504  alpha_Isc=0.0030079  IL=6.4137  I0=6.5578e-13  nI=0.95237  Rsh=7.312  Rs=0.0042689  RobustModel=on  RobustCellTemperature=25  BAL=on  Tc=1e-5  Tfilter=5e-5
  Terminator1 : Terminator
  Variable Resistor2 : spsVariableResistorLib/Variable Resistor  Rabsmin=1e-3
      settings: LibrarySourceBlock=sps_lib/Passives/Variable Resistor
  + : PMIOPort  Side=Left
  - : PMIOPort  Port=2  Side=Right
  wires:
  Irr/1 -> PV2/1
  1PΩ/1 -> Variable Resistor2/1
  PV2/1 -> Terminator1/1
  connections:
  -/RConn1 -- PV2/RConn2 -- Variable Resistor2/RConn1
  +/RConn1 -- PV2/RConn1 -- Variable Resistor2/LConn1

== system String3_Diode/Subsystem36/PV4 ==
  Irr : Inport
  1PΩ : Constant  Value=1e15
  PV2 : spsPVArrayLib/PV Array  Npar=1  Nser=1  PlotType=array @ 25 deg.C & specified irradiances  S_vec="[ 1000  500  100 ]"  Temp_C_vec="[ 45 25  ]"  ModuleName=User-defined  PlotWhenSelected=off  Pm=3.8061  Ncell=1  Voc=0.7315  Isc=6.41  Vm=0.626  Im=6.08  beta_Voc_pc=-0.2256195755  alpha_Isc_pc=0.04692556634  beta_Voc=-0.0016504  alpha_Isc=0.0030079  IL=6.4137  I0=6.5578e-13  nI=0.95237  Rsh=7.312  Rs=0.0042689  RobustModel=on  RobustCellTemperature=25  BAL=on  Tc=1e-5  Tfilter=5e-5
  Terminator1 : Terminator
  Variable Resistor2 : spsVariableResistorLib/Variable Resistor  Rabsmin=1e-3
      settings: LibrarySourceBlock=sps_lib/Passives/Variable Resistor
  + : PMIOPort  Side=Left
  - : PMIOPort  Port=2  Side=Right
  wires:
  Irr/1 -> PV2/1
  1PΩ/1 -> Variable Resistor2/1
  PV2/1 -> Terminator1/1
  connections:
  -/RConn1 -- Variable Resistor2/RConn1 -- PV2/RConn2
  +/RConn1 -- Variable Resistor2/LConn1 -- PV2/RConn1

== system String3_Diode/Subsystem37/PV1 ==
  Irr : Inport
  1PΩ : Constant  Value=1e15
  PV2 : spsPVArrayLib/PV Array  Npar=1  Nser=1  PlotType=array @ 25 deg.C & specified irradiances  S_vec="[ 1000  500  100 ]"  Temp_C_vec="[ 45 25  ]"  ModuleName=User-defined  PlotWhenSelected=off  Pm=3.8061  Ncell=1  Voc=0.7315  Isc=6.41  Vm=0.626  Im=6.08  beta_Voc_pc=-0.2256195755  alpha_Isc_pc=0.04692556634  beta_Voc=-0.0016504  alpha_Isc=0.0030079  IL=6.4137  I0=6.5578e-13  nI=0.95237  Rsh=7.312  Rs=0.0042689  RobustModel=on  RobustCellTemperature=25  BAL=on  Tc=1e-5  Tfilter=5e-5
  Terminator1 : Terminator
  Variable Resistor2 : spsVariableResistorLib/Variable Resistor  Rabsmin=1e-3
      settings: LibrarySourceBlock=sps_lib/Passives/Variable Resistor
  + : PMIOPort  Side=Left
  - : PMIOPort  Port=2  Side=Right
  wires:
  Irr/1 -> PV2/1
  1PΩ/1 -> Variable Resistor2/1
  PV2/1 -> Terminator1/1
  connections:
  -/RConn1 -- Variable Resistor2/RConn1 -- PV2/RConn2
  +/RConn1 -- Variable Resistor2/LConn1 -- PV2/RConn1

== system String3_Diode/Subsystem37/PV2 ==
  Irr : Inport
  1PΩ : Constant  Value=1e15
  PV2 : spsPVArrayLib/PV Array  Npar=1  Nser=1  PlotType=array @ 25 deg.C & specified irradiances  S_vec="[ 1000  500  100 ]"  Temp_C_vec="[ 45 25  ]"  ModuleName=User-defined  PlotWhenSelected=off  Pm=3.8061  Ncell=1  Voc=0.7315  Isc=6.41  Vm=0.626  Im=6.08  beta_Voc_pc=-0.2256195755  alpha_Isc_pc=0.04692556634  beta_Voc=-0.0016504  alpha_Isc=0.0030079  IL=6.4137  I0=6.5578e-13  nI=0.95237  Rsh=7.312  Rs=0.0042689  RobustModel=on  RobustCellTemperature=25  BAL=on  Tc=1e-5  Tfilter=5e-5
  Terminator1 : Terminator
  Variable Resistor2 : spsVariableResistorLib/Variable Resistor  Rabsmin=1e-3
      settings: LibrarySourceBlock=sps_lib/Passives/Variable Resistor
  + : PMIOPort  Side=Left
  - : PMIOPort  Port=2  Side=Right
  wires:
  Irr/1 -> PV2/1
  1PΩ/1 -> Variable Resistor2/1
  PV2/1 -> Terminator1/1
  connections:
  -/RConn1 -- Variable Resistor2/RConn1 -- PV2/RConn2
  +/RConn1 -- Variable Resistor2/LConn1 -- PV2/RConn1

== system String3_Diode/Subsystem37/PV3 ==
  Irr : Inport
  1PΩ : Constant  Value=1e15
  PV2 : spsPVArrayLib/PV Array  Npar=1  Nser=1  PlotType=array @ 25 deg.C & specified irradiances  S_vec="[ 1000  500  100 ]"  Temp_C_vec="[ 45 25  ]"  ModuleName=User-defined  PlotWhenSelected=off  Pm=3.8061  Ncell=1  Voc=0.7315  Isc=6.41  Vm=0.626  Im=6.08  beta_Voc_pc=-0.2256195755  alpha_Isc_pc=0.04692556634  beta_Voc=-0.0016504  alpha_Isc=0.0030079  IL=6.4137  I0=6.5578e-13  nI=0.95237  Rsh=7.312  Rs=0.0042689  RobustModel=on  RobustCellTemperature=25  BAL=on  Tc=1e-5  Tfilter=5e-5
  Terminator1 : Terminator
  Variable Resistor2 : spsVariableResistorLib/Variable Resistor  Rabsmin=1e-3
      settings: LibrarySourceBlock=sps_lib/Passives/Variable Resistor
  + : PMIOPort  Side=Left
  - : PMIOPort  Port=2  Side=Right
  wires:
  Irr/1 -> PV2/1
  1PΩ/1 -> Variable Resistor2/1
  PV2/1 -> Terminator1/1
  connections:
  -/RConn1 -- PV2/RConn2 -- Variable Resistor2/RConn1
  +/RConn1 -- PV2/RConn1 -- Variable Resistor2/LConn1

== system String3_Diode/Subsystem37/PV4 ==
  Irr : Inport
  1PΩ : Constant  Value=1e15
  PV2 : spsPVArrayLib/PV Array  Npar=1  Nser=1  PlotType=array @ 25 deg.C & specified irradiances  S_vec="[ 1000  500  100 ]"  Temp_C_vec="[ 45 25  ]"  ModuleName=User-defined  PlotWhenSelected=off  Pm=3.8061  Ncell=1  Voc=0.7315  Isc=6.41  Vm=0.626  Im=6.08  beta_Voc_pc=-0.2256195755  alpha_Isc_pc=0.04692556634  beta_Voc=-0.0016504  alpha_Isc=0.0030079  IL=6.4137  I0=6.5578e-13  nI=0.95237  Rsh=7.312  Rs=0.0042689  RobustModel=on  RobustCellTemperature=25  BAL=on  Tc=1e-5  Tfilter=5e-5
  Terminator1 : Terminator
  Variable Resistor2 : spsVariableResistorLib/Variable Resistor  Rabsmin=1e-3
      settings: LibrarySourceBlock=sps_lib/Passives/Variable Resistor
  + : PMIOPort  Side=Left
  - : PMIOPort  Port=2  Side=Right
  wires:
  Irr/1 -> PV2/1
  1PΩ/1 -> Variable Resistor2/1
  PV2/1 -> Terminator1/1
  connections:
  -/RConn1 -- Variable Resistor2/RConn1 -- PV2/RConn2
  +/RConn1 -- Variable Resistor2/LConn1 -- PV2/RConn1

== system String3_Diode/Subsystem38/PV1 ==
  Irr : Inport
  1PΩ : Constant  Value=1e15
  PV2 : spsPVArrayLib/PV Array  Npar=1  Nser=1  PlotType=array @ 25 deg.C & specified irradiances  S_vec="[ 1000  500  100 ]"  Temp_C_vec="[ 45 25  ]"  ModuleName=User-defined  PlotWhenSelected=off  Pm=3.8061  Ncell=1  Voc=0.7315  Isc=6.41  Vm=0.626  Im=6.08  beta_Voc_pc=-0.2256195755  alpha_Isc_pc=0.04692556634  beta_Voc=-0.0016504  alpha_Isc=0.0030079  IL=6.4137  I0=6.5578e-13  nI=0.95237  Rsh=7.312  Rs=0.0042689  RobustModel=on  RobustCellTemperature=25  BAL=on  Tc=1e-5  Tfilter=5e-5
  Terminator1 : Terminator
  Variable Resistor2 : spsVariableResistorLib/Variable Resistor  Rabsmin=1e-3
      settings: LibrarySourceBlock=sps_lib/Passives/Variable Resistor
  + : PMIOPort  Side=Left
  - : PMIOPort  Port=2  Side=Right
  wires:
  Irr/1 -> PV2/1
  1PΩ/1 -> Variable Resistor2/1
  PV2/1 -> Terminator1/1
  connections:
  -/RConn1 -- Variable Resistor2/RConn1 -- PV2/RConn2
  +/RConn1 -- Variable Resistor2/LConn1 -- PV2/RConn1

== system String3_Diode/Subsystem38/PV2 ==
  Irr : Inport
  1PΩ : Constant  Value=1e15
  PV2 : spsPVArrayLib/PV Array  Npar=1  Nser=1  PlotType=array @ 25 deg.C & specified irradiances  S_vec="[ 1000  500  100 ]"  Temp_C_vec="[ 45 25  ]"  ModuleName=User-defined  PlotWhenSelected=off  Pm=3.8061  Ncell=1  Voc=0.7315  Isc=6.41  Vm=0.626  Im=6.08  beta_Voc_pc=-0.2256195755  alpha_Isc_pc=0.04692556634  beta_Voc=-0.0016504  alpha_Isc=0.0030079  IL=6.4137  I0=6.5578e-13  nI=0.95237  Rsh=7.312  Rs=0.0042689  RobustModel=on  RobustCellTemperature=25  BAL=on  Tc=1e-5  Tfilter=5e-5
  Terminator1 : Terminator
  Variable Resistor2 : spsVariableResistorLib/Variable Resistor  Rabsmin=1e-3
      settings: LibrarySourceBlock=sps_lib/Passives/Variable Resistor
  + : PMIOPort  Side=Left
  - : PMIOPort  Port=2  Side=Right
  wires:
  Irr/1 -> PV2/1
  1PΩ/1 -> Variable Resistor2/1
  PV2/1 -> Terminator1/1
  connections:
  -/RConn1 -- Variable Resistor2/RConn1 -- PV2/RConn2
  +/RConn1 -- Variable Resistor2/LConn1 -- PV2/RConn1

== system String3_Diode/Subsystem38/PV3 ==
  Irr : Inport
  1PΩ : Constant  Value=1e15
  PV2 : spsPVArrayLib/PV Array  Npar=1  Nser=1  PlotType=array @ 25 deg.C & specified irradiances  S_vec="[ 1000  500  100 ]"  Temp_C_vec="[ 45 25  ]"  ModuleName=User-defined  PlotWhenSelected=off  Pm=3.8061  Ncell=1  Voc=0.7315  Isc=6.41  Vm=0.626  Im=6.08  beta_Voc_pc=-0.2256195755  alpha_Isc_pc=0.04692556634  beta_Voc=-0.0016504  alpha_Isc=0.0030079  IL=6.4137  I0=6.5578e-13  nI=0.95237  Rsh=7.312  Rs=0.0042689  RobustModel=on  RobustCellTemperature=25  BAL=on  Tc=1e-5  Tfilter=5e-5
  Terminator1 : Terminator
  Variable Resistor2 : spsVariableResistorLib/Variable Resistor  Rabsmin=1e-3
      settings: LibrarySourceBlock=sps_lib/Passives/Variable Resistor
  + : PMIOPort  Side=Left
  - : PMIOPort  Port=2  Side=Right
  wires:
  Irr/1 -> PV2/1
  1PΩ/1 -> Variable Resistor2/1
  PV2/1 -> Terminator1/1
  connections:
  -/RConn1 -- PV2/RConn2 -- Variable Resistor2/RConn1
  +/RConn1 -- PV2/RConn1 -- Variable Resistor2/LConn1

== system String3_Diode/Subsystem38/PV4 ==
  Irr : Inport
  1PΩ : Constant  Value=1e15
  PV2 : spsPVArrayLib/PV Array  Npar=1  Nser=1  PlotType=array @ 25 deg.C & specified irradiances  S_vec="[ 1000  500  100 ]"  Temp_C_vec="[ 45 25  ]"  ModuleName=User-defined  PlotWhenSelected=off  Pm=3.8061  Ncell=1  Voc=0.7315  Isc=6.41  Vm=0.626  Im=6.08  beta_Voc_pc=-0.2256195755  alpha_Isc_pc=0.04692556634  beta_Voc=-0.0016504  alpha_Isc=0.0030079  IL=6.4137  I0=6.5578e-13  nI=0.95237  Rsh=7.312  Rs=0.0042689  RobustModel=on  RobustCellTemperature=25  BAL=on  Tc=1e-5  Tfilter=5e-5
  Terminator1 : Terminator
  Variable Resistor2 : spsVariableResistorLib/Variable Resistor  Rabsmin=1e-3
      settings: LibrarySourceBlock=sps_lib/Passives/Variable Resistor
  + : PMIOPort  Side=Left
  - : PMIOPort  Port=2  Side=Right
  wires:
  Irr/1 -> PV2/1
  1PΩ/1 -> Variable Resistor2/1
  PV2/1 -> Terminator1/1
  connections:
  -/RConn1 -- Variable Resistor2/RConn1 -- PV2/RConn2
  +/RConn1 -- Variable Resistor2/LConn1 -- PV2/RConn1

== system String3_Diode/Subsystem39/PV1 ==
  Irr : Inport
  1PΩ : Constant  Value=1e15
  PV2 : spsPVArrayLib/PV Array  Npar=1  Nser=1  PlotType=array @ 25 deg.C & specified irradiances  S_vec="[ 1000  500  100 ]"  Temp_C_vec="[ 45 25  ]"  ModuleName=User-defined  PlotWhenSelected=off  Pm=3.8061  Ncell=1  Voc=0.7315  Isc=6.41  Vm=0.626  Im=6.08  beta_Voc_pc=-0.2256195755  alpha_Isc_pc=0.04692556634  beta_Voc=-0.0016504  alpha_Isc=0.0030079  IL=6.4137  I0=6.5578e-13  nI=0.95237  Rsh=7.312  Rs=0.0042689  RobustModel=on  RobustCellTemperature=25  BAL=on  Tc=1e-5  Tfilter=5e-5
  Terminator1 : Terminator
  Variable Resistor2 : spsVariableResistorLib/Variable Resistor  Rabsmin=1e-3
      settings: LibrarySourceBlock=sps_lib/Passives/Variable Resistor
  + : PMIOPort  Side=Left
  - : PMIOPort  Port=2  Side=Right
  wires:
  Irr/1 -> PV2/1
  1PΩ/1 -> Variable Resistor2/1
  PV2/1 -> Terminator1/1
  connections:
  -/RConn1 -- Variable Resistor2/RConn1 -- PV2/RConn2
  +/RConn1 -- Variable Resistor2/LConn1 -- PV2/RConn1

== system String3_Diode/Subsystem39/PV2 ==
  Irr : Inport
  1PΩ : Constant  Value=1e15
  PV2 : spsPVArrayLib/PV Array  Npar=1  Nser=1  PlotType=array @ 25 deg.C & specified irradiances  S_vec="[ 1000  500  100 ]"  Temp_C_vec="[ 45 25  ]"  ModuleName=User-defined  PlotWhenSelected=off  Pm=3.8061  Ncell=1  Voc=0.7315  Isc=6.41  Vm=0.626  Im=6.08  beta_Voc_pc=-0.2256195755  alpha_Isc_pc=0.04692556634  beta_Voc=-0.0016504  alpha_Isc=0.0030079  IL=6.4137  I0=6.5578e-13  nI=0.95237  Rsh=7.312  Rs=0.0042689  RobustModel=on  RobustCellTemperature=25  BAL=on  Tc=1e-5  Tfilter=5e-5
  Terminator1 : Terminator
  Variable Resistor2 : spsVariableResistorLib/Variable Resistor  Rabsmin=1e-3
      settings: LibrarySourceBlock=sps_lib/Passives/Variable Resistor
  + : PMIOPort  Side=Left
  - : PMIOPort  Port=2  Side=Right
  wires:
  Irr/1 -> PV2/1
  1PΩ/1 -> Variable Resistor2/1
  PV2/1 -> Terminator1/1
  connections:
  -/RConn1 -- Variable Resistor2/RConn1 -- PV2/RConn2
  +/RConn1 -- Variable Resistor2/LConn1 -- PV2/RConn1

== system String3_Diode/Subsystem39/PV3 ==
  Irr : Inport
  1PΩ : Constant  Value=1e15
  PV2 : spsPVArrayLib/PV Array  Npar=1  Nser=1  PlotType=array @ 25 deg.C & specified irradiances  S_vec="[ 1000  500  100 ]"  Temp_C_vec="[ 45 25  ]"  ModuleName=User-defined  PlotWhenSelected=off  Pm=3.8061  Ncell=1  Voc=0.7315  Isc=6.41  Vm=0.626  Im=6.08  beta_Voc_pc=-0.2256195755  alpha_Isc_pc=0.04692556634  beta_Voc=-0.0016504  alpha_Isc=0.0030079  IL=6.4137  I0=6.5578e-13  nI=0.95237  Rsh=7.312  Rs=0.0042689  RobustModel=on  RobustCellTemperature=25  BAL=on  Tc=1e-5  Tfilter=5e-5
  Terminator1 : Terminator
  Variable Resistor2 : spsVariableResistorLib/Variable Resistor  Rabsmin=1e-3
      settings: LibrarySourceBlock=sps_lib/Passives/Variable Resistor
  + : PMIOPort  Side=Left
  - : PMIOPort  Port=2  Side=Right
  wires:
  Irr/1 -> PV2/1
  1PΩ/1 -> Variable Resistor2/1
  PV2/1 -> Terminator1/1
  connections:
  -/RConn1 -- PV2/RConn2 -- Variable Resistor2/RConn1
  +/RConn1 -- PV2/RConn1 -- Variable Resistor2/LConn1

== system String3_Diode/Subsystem39/PV4 ==
  Irr : Inport
  1PΩ : Constant  Value=1e15
  PV2 : spsPVArrayLib/PV Array  Npar=1  Nser=1  PlotType=array @ 25 deg.C & specified irradiances  S_vec="[ 1000  500  100 ]"  Temp_C_vec="[ 45 25  ]"  ModuleName=User-defined  PlotWhenSelected=off  Pm=3.8061  Ncell=1  Voc=0.7315  Isc=6.41  Vm=0.626  Im=6.08  beta_Voc_pc=-0.2256195755  alpha_Isc_pc=0.04692556634  beta_Voc=-0.0016504  alpha_Isc=0.0030079  IL=6.4137  I0=6.5578e-13  nI=0.95237  Rsh=7.312  Rs=0.0042689  RobustModel=on  RobustCellTemperature=25  BAL=on  Tc=1e-5  Tfilter=5e-5
  Terminator1 : Terminator
  Variable Resistor2 : spsVariableResistorLib/Variable Resistor  Rabsmin=1e-3
      settings: LibrarySourceBlock=sps_lib/Passives/Variable Resistor
  + : PMIOPort  Side=Left
  - : PMIOPort  Port=2  Side=Right
  wires:
  Irr/1 -> PV2/1
  1PΩ/1 -> Variable Resistor2/1
  PV2/1 -> Terminator1/1
  connections:
  -/RConn1 -- Variable Resistor2/RConn1 -- PV2/RConn2
  +/RConn1 -- Variable Resistor2/LConn1 -- PV2/RConn1

== system String3_Diode/Subsystem4/PV1 ==
  Irr : Inport
  1PΩ : Constant  Value=1e15
  PV2 : spsPVArrayLib/PV Array  Npar=1  Nser=1  PlotType=array @ 25 deg.C & specified irradiances  S_vec="[ 1000  500  100 ]"  Temp_C_vec="[ 45 25  ]"  ModuleName=User-defined  PlotWhenSelected=off  Pm=3.8061  Ncell=1  Voc=0.7315  Isc=6.41  Vm=0.626  Im=6.08  beta_Voc_pc=-0.2256195755  alpha_Isc_pc=0.04692556634  beta_Voc=-0.0016504  alpha_Isc=0.0030079  IL=6.4137  I0=6.5578e-13  nI=0.95237  Rsh=7.312  Rs=0.0042689  RobustModel=on  RobustCellTemperature=25  BAL=on  Tc=1e-5  Tfilter=5e-5
  Terminator1 : Terminator
  Variable Resistor2 : spsVariableResistorLib/Variable Resistor  Rabsmin=1e-3
      settings: LibrarySourceBlock=sps_lib/Passives/Variable Resistor
  + : PMIOPort  Side=Left
  - : PMIOPort  Port=2  Side=Right
  wires:
  Irr/1 -> PV2/1
  1PΩ/1 -> Variable Resistor2/1
  PV2/1 -> Terminator1/1
  connections:
  -/RConn1 -- Variable Resistor2/RConn1 -- PV2/RConn2
  +/RConn1 -- Variable Resistor2/LConn1 -- PV2/RConn1

== system String3_Diode/Subsystem4/PV10 ==
  Irr : Inport
  1PΩ : Constant  Value=1e15
  PV1 : spsPVArrayLib/PV Array  Npar=1  Nser=1  PlotType=array @ 25 deg.C & specified irradiances  S_vec="[ 1000  500  100 ]"  Temp_C_vec="[ 45 25  ]"  ModuleName=User-defined  PlotWhenSelected=off  Pm=3.8061  Ncell=1  Voc=0.7315  Isc=6.41  Vm=0.626  Im=6.08  beta_Voc_pc=-0.2256195755  alpha_Isc_pc=0.04692556634  beta_Voc=-0.0016504  alpha_Isc=0.0030079  IL=6.4137  I0=6.5578e-13  nI=0.95237  Rsh=7.312  Rs=0.0042689  RobustModel=on  RobustCellTemperature=25  BAL=on  Tc=1e-5  Tfilter=5e-5
  Terminator1 : Terminator
  Variable Resistor2 : spsVariableResistorLib/Variable Resistor  Rabsmin=1e-3
      settings: LibrarySourceBlock=sps_lib/Passives/Variable Resistor
  + : PMIOPort  Side=Left
  - : PMIOPort  Port=2  Side=Right
  wires:
  Irr/1 -> PV1/1
  1PΩ/1 -> Variable Resistor2/1
  PV1/1 -> Terminator1/1
  connections:
  PV1/RConn2 -- -/RConn1 -- Variable Resistor2/RConn1
  +/RConn1 -- Variable Resistor2/LConn1 -- PV1/RConn1

== system String3_Diode/Subsystem4/PV11 ==
  Irr : Inport
  1PΩ : Constant  Value=1e15
  PV2 : spsPVArrayLib/PV Array  Npar=1  Nser=1  PlotType=array @ 25 deg.C & specified irradiances  S_vec="[ 1000  500  100 ]"  Temp_C_vec="[ 45 25  ]"  ModuleName=User-defined  PlotWhenSelected=off  Pm=3.8061  Ncell=1  Voc=0.7315  Isc=6.41  Vm=0.626  Im=6.08  beta_Voc_pc=-0.2256195755  alpha_Isc_pc=0.04692556634  beta_Voc=-0.0016504  alpha_Isc=0.0030079  IL=6.4137  I0=6.5578e-13  nI=0.95237  Rsh=7.312  Rs=0.0042689  RobustModel=on  RobustCellTemperature=25  BAL=on  Tc=1e-5  Tfilter=5e-5
  Terminator1 : Terminator
  Variable Resistor2 : spsVariableResistorLib/Variable Resistor  Rabsmin=1e-3
      settings: LibrarySourceBlock=sps_lib/Passives/Variable Resistor
  + : PMIOPort  Side=Left
  - : PMIOPort  Port=2  Side=Right
  wires:
  Irr/1 -> PV2/1
  1PΩ/1 -> Variable Resistor2/1
  PV2/1 -> Terminator1/1
  connections:
  -/RConn1 -- Variable Resistor2/RConn1 -- PV2/RConn2
  +/RConn1 -- Variable Resistor2/LConn1 -- PV2/RConn1
